simulink model "testing"  (R2023a)
settings: Solver=VariableStepAuto  StartTime=0.0  StopTime=50  RelTol=1e-3
libraries: hdlsllib x2, dsphdlxfrm2 x1, commutil2 x1
settings Model: NumberOfSteps=5  Creator=acer  LastModifiedBy=acer
settings OptimizationCC: BlockReduction=off  ConditionallyExecuteInputs=off

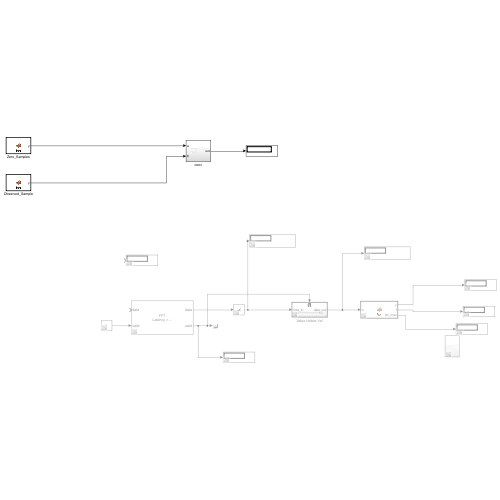
[thumbnail: Simulink's stored preview of the top-level diagram]
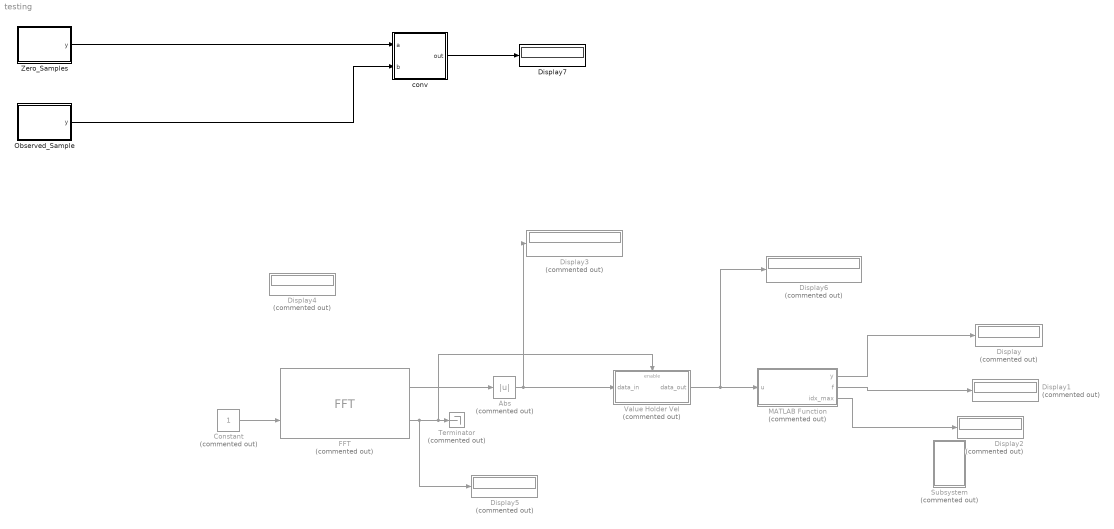
== system testing ==
  Abs : Abs  Commented=on  SaturateOnIntegerOverflow=off
  Constant : Constant  Commented=on  OutDataTypeStr=boolean  SampleTime=-1
  Display{,1..6} (7 alike) : Display  Commented=on
  Display7 : Display
  FFT : dsphdlxfrm2/FFT  Commented=on  FFTLength=32  Architecture=Streaming Radix 2^2  ComplexMultiplication=Use 4 multipliers and 2 adders  BitReversedOutput=on  BitReversedInput=off  Normalize=off  SimulateUsing=Code generation  RoundingMethod=Floor  ResetInputPort=off  StartOutputPort=off  EndOutputPort=off
  MATLAB Function : MATLAB Function  Commented=on  TreatAsAtomicUnit=on
  Observed_Sample : MATLAB Function  TreatAsAtomicUnit=on
  Subsystem : Subsystem  Commented=on
  Terminator : Terminator  Commented=on
  Value Holder Vel : Subsystem  Commented=on  TreatAsAtomicUnit=on
      settings: LibrarySourceBlock=|
      | hdlsllib/Ports &
      | Subsystems/Enabled
      | Subsystem
  Zero_Samples : MATLAB Function  TreatAsAtomicUnit=on
  conv : Subsystem
  wires:
  Constant/1 -> FFT/2
  FFT/2 -> Display5/1, Value Holder Vel/Enable, Terminator/1
  FFT/1 -> Abs/1
  Abs/1 -> Value Holder Vel/1(data_in), Display3/1
  MATLAB Function/1(y) -> Display/1
  MATLAB Function/2(f) -> Display1/1
  MATLAB Function/3(idx_max) -> Display2/1
  Value Holder Vel/1(data_out) -> Display6/1, MATLAB Function/1(u)
  Zero_Samples/1(y) -> conv/1(a)
  Observed_Sample/1(y) -> conv/2(b)
  conv/1(out) -> Display7/1

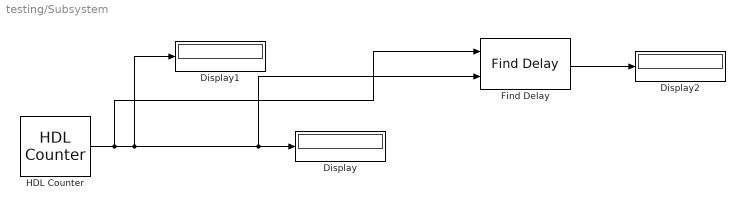
== system testing/Subsystem ==
  Display : Display
  Display1 : Display
  Display2 : Display
  Find Delay : commutil2/Find Delay  corrLength=200  chgSigOP=off  stopUpdate=off  numConstDelay=3
  HDL Counter : hdlsllib/Sources/HDL Counter  CountType=Count limited  CountInit=0  CountStep=1  CountMax=25  CountFromType=Initial value  CountFrom=0  CountResetPort=off  CountLoadPort=off  CountEnbPort=off  CountDirPort=off  CountHitOutputPort=off  CountDataType=Unsigned  CountWordLen=8  CountFracLen=0  CountSampTime=1
  wires:
  Find Delay/1 -> Display2/1
  HDL Counter/1 -> Find Delay/1, Find Delay/2, Display/1, Display1/1

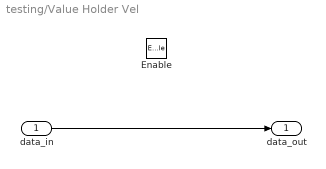
== system testing/Value Holder Vel ==
  data_in : Inport
  Enable : EnablePort
  data_out : Outport  InitialOutput=0
  wires:
  data_in/1 -> data_out/1

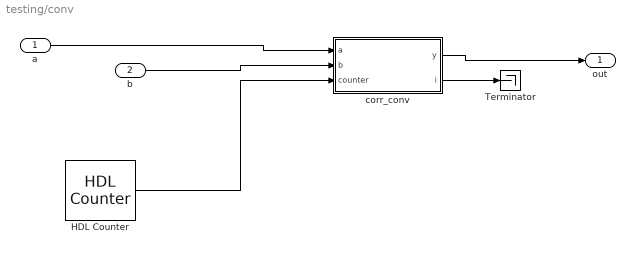
== system testing/conv ==
  a : Inport  OutMin=0  OutMax=1  OutDataTypeStr=fixdt(1,16)
  b : Inport  Port=2  OutMin=0  OutMax=1  OutDataTypeStr=fixdt(1,12)
  HDL Counter : hdlsllib/Sources/HDL Counter  CountType=Count limited  CountInit=0  CountStep=1  CountMax=25  CountFromType=Initial value  CountFrom=0  CountResetPort=off  CountLoadPort=off  CountEnbPort=off  CountDirPort=off  CountHitOutputPort=off  CountDataType=Unsigned  CountWordLen=8  CountFracLen=0  CountSampTime=1e-5
  Terminator : Terminator
  corr_conv : MATLAB Function  TreatAsAtomicUnit=on
  out : Outport
  wires:
  corr_conv/1(y) -> out/1
  a/1 -> corr_conv/1(a)
  b/1 -> corr_conv/2(b)
  corr_conv/2(i) -> Terminator/1
  HDL Counter/1 -> corr_conv/3(counter)

== matlab function testing/Zero_Samples ==
  data: y output
function y = fcn()
%#codegen

rx_signal = fi(zeros(32,1),1,16,14);

y = rx_signal;

== matlab function testing/MATLAB Function ==
  data: u input; y output; f output; idx_max output
function [y,f,idx_max] = fcn(u)
%#codegen

N = uint16(length(u)/2);
max = 0;
idx_max = uint16(0);

for i=1:N/2
    if(u(i) > max )
        max = u(i);
        idx_max = i;
    end
end

f = fi(idx_max * 5000 / (N*2),0,32,5);

y = f * 0.1 / 2;

== matlab function testing/conv/corr_conv ==
  data: a input; y output; b input; i output; counter input
function [y,i] = fcn(a,b, counter)
%#codegen

if(counter >= 5)
    yy = conv(a,flipud(b));
    size_yy =  uint16(size(yy, 1));
    yy_idxes = uint16(1:round(size_yy/2));
    yy_abs = (yy(round(size_yy/2):size_yy,1));
    
    max_yy = max(yy_abs);
    max_idx = uint16(0);

    % for i=yy_idxes
    %     if(yy(i) >= max_yy)
    %         max_yy = yy(i);
    %         max_idx = i;
    %     end
    % end
    y = max_yy;
    i = max_idx;
else
    y = fi(0,1,33,24);
    i = uint16(0);
end


% i = uint16(lag_of_max_yy);

== matlab function testing/Observed_Sample ==
  data: y output
function y = fcn()
%#codegen

rx_signal = [
4.06834681001246e-05
8.69706183656938e-05
0.000106025085684376
-3.68060079828934e-05
-3.09338181300556e-05
-5.80614437815797e-05
4.16482966649317e-05
-2.64609700338026e-05
-0.000137751663330026
7.66747644261270e-06
0
0
0
0
0
0
0
0
0
0
0
0
0
0
0
0
0
0
0
0
0
0];

y = fi(rx_signal,1,12,10);
